simulink model "project2"  (R2020b)
settings: Solver=VariableStepAuto  StartTime=0.0  StopTime=10.0  RelTol=1e-3
model workspace (MAT data in the model file):
  M1 = 100
  M2 = 4
  b = 50
  k1 = 50
  k2 = 25
settings Model: ParameterArgumentNames=b  OrderedModelArguments=off  Creator=admin  LastModifiedBy=admin

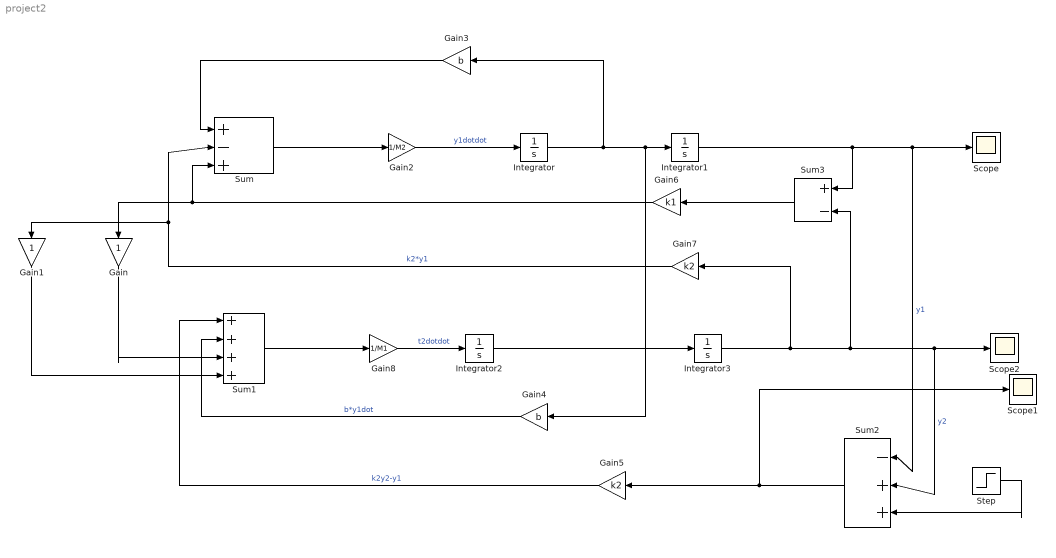
== system project2 ==
  Gain : Gain
  Gain1 : Gain
  Gain2 : Gain  Gain=1/M2
  Gain3 : Gain  Gain=b
  Gain4 : Gain  Gain=b
  Gain5 : Gain  Gain=k2
  Gain6 : Gain  Gain=k1
  Gain7 : Gain  Gain=k2
  Gain8 : Gain  Gain=1/M1
  Integrator{,1..3} (4 alike) : Integrator
  Scope : Scope
  Scope1 : Scope
  Scope2 : Scope
  Step : Step  SampleTime=0
  Sum : Sum  Inputs=|+-+
  Sum1 : Sum  Inputs=|++++
  Sum2 : Sum  Inputs=|-++
  Sum3 : Sum  Inputs=+-
  wires:
  Sum/1 -> Gain2/1
  Gain2/1 -> Integrator/1  "y1dotdot"
  Integrator/1 -> Gain3/1, Gain4/1, Integrator1/1
  Sum1/1 -> Gain8/1
  Gain8/1 -> Integrator2/1  "t2dotdot"
  Integrator2/1 -> Integrator3/1
  Gain3/1 -> Sum/1
  Gain7/1 -> Gain1/1, Sum/2  "k2*y1"
  Gain1/1 -> Sum1/4
  Gain/1 -> Sum1/3
  Gain4/1 -> Sum1/2  "b*y1dot"
  Gain5/1 -> Sum1/1  "k2y2-y1"
  Sum2/1 -> Scope1/1, Gain5/1
  Sum3/1 -> Gain6/1
  Integrator3/1 -> Gain7/1, Sum3/2, Sum2/2, Scope2/1  "y2"
  Step/1 -> Sum2/3
  Integrator1/1 -> Sum2/1, Scope/1, Sum3/1  "y1"
  Gain6/1 -> Sum/3, Gain/1
